simulink model "simulation_nonscalar"  (R2021b)
settings: Solver=VariableStepAuto  StartTime=0.0  StopTime=3  MaxStep=0.005  RelTol=1e-3
values from neighbouring files (symbols this model uses):
  A = round(A,1)    [nonscalar_net.m]    (also in scalar.mat = [-1.7 0 0 0 0 0 -4.8 0 0 0 0 0 ... (25 elements, 5x5)]; scalar_net.m; scalar_net_CreationNewConnection.m = diag([-1,-3,-2]); scalar_net_exception1.m)
  M = [-1.5 0 -0.7 0 17.9 0 -4.1 -6.8 0 0 0 0 ... (25 elements, 5x5)]    [exception.mat]    (also in nonscalar.mat = [-3.8 1.9 -4.5 0 0 0 -4.6 1.6 0 0 0 0 ... (25 elements, 5x5); nonscalar_net.m = round(M,1); nonscalar_net_general.m = sym('M',sum(n)); robustness.mat = [-8.5 0 -1.6 0 1.5 0 -5.3 -4.7 0 0 0 0 ... (25 elements, 5x5)
  M_bar = [-8.5 0 -1.6 0 2.22044604925e-16 0 -5.3 -4.7 0 0 0 0 ... (25 elements, 5x5)]    [robustness.mat]    (also in scalar.mat = [-1.7 0 -6.4 0 0.05 0 -4.8 -9.5 0 0 0 0 ... (25 elements, 5x; test_meerkov_nonscalar_different.m = M + B_bar; test_meerkov_nonscalar_equal.m = M + V_bar)
  mu = sqrt(abs(2/(M(4,5)*M(5,4))))*omega    [nonscalar_net.m]
  n = 1    [exception.mat]    (also in nonscalar_net.m = [1,3,1]; nonscalar_net_general.m = [1,1,1,1]; random.m; robustness.mat)
  omega = 200    [nonscalar.mat]    (also in nonscalar_net.m = 50)
  x_0 = [1 1 1 1 1]    [exception.mat]    (also in nonscalar_net.m = ones(sum(n),1); robustness.mat; scalar.mat; scalar_net.m = ones(5,1))
  y_0 = double(inv_F0*x_0)    [nonscalar_net.m]    (also in scalar_net.m)
settings Model: Creator=alber  LastModifiedBy=alber

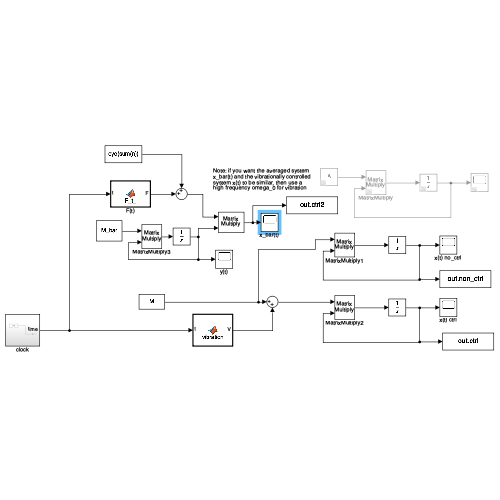
[thumbnail: Simulink's stored preview of the top-level diagram]
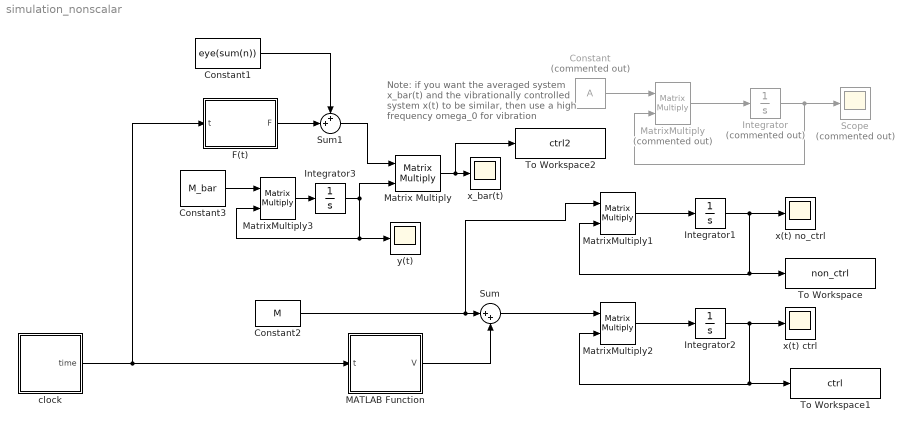
== system simulation_nonscalar ==
  note: Note: if you want the averaged system x_bar(t) and the vibrationally controlled system x(t) to be similar, then use a high frequency omega_0 for vibration
  Constant : Constant  Commented=on  Value=A
  Constant1 : Constant  Value=eye(sum(n))
  Constant2 : Constant  Value=M
  Constant3 : Constant  Value=M_bar
  F(t) : MATLAB Function  TreatAsAtomicUnit=on
  Integrator : Integrator  Commented=on  InitialCondition=x_0
  Integrator1 : Integrator  InitialCondition=x_0
  Integrator2 : Integrator  InitialCondition=x_0
  Integrator3 : Integrator  InitialCondition=y_0
  MATLAB Function : MATLAB Function  TreatAsAtomicUnit=on
  Matrix Multiply : Product  Multiplication=Matrix(*)
  MatrixMultiply : Product  Commented=on  Multiplication=Matrix(*)
  MatrixMultiply1 : Product  Multiplication=Matrix(*)
  MatrixMultiply2 : Product  Multiplication=Matrix(*)
  MatrixMultiply3 : Product  Multiplication=Matrix(*)
  Scope : Scope  Commented=on
  Sum : Sum  Inputs=|++
  Sum1 : Sum  Inputs=++|
  To Workspace : ToWorkspace  VariableName=non_ctrl  SaveFormat=Timeseries  SampleTime=-1
  To Workspace1 : ToWorkspace  VariableName=ctrl  SaveFormat=Timeseries  SampleTime=-1
  To Workspace2 : ToWorkspace  VariableName=ctrl2  SaveFormat=Timeseries  SampleTime=-1
  clock : Subsystem
  x(t) ctrl : Scope
  x(t) no_ctrl : Scope
  x_bar(t) : Scope
  y(t) : Scope
  wires:
  Constant/1 -> MatrixMultiply/1
  Integrator/1 -> Scope/1, MatrixMultiply/2
  MatrixMultiply/1 -> Integrator/1
  MatrixMultiply1/1 -> Integrator1/1
  Constant2/1 -> MatrixMultiply1/1, Sum/1
  Integrator1/1 -> x(t) no_ctrl/1, MatrixMultiply1/2, To Workspace/1
  Integrator2/1 -> x(t) ctrl/1, To Workspace1/1, MatrixMultiply2/2
  MatrixMultiply2/1 -> Integrator2/1
  Sum/1 -> MatrixMultiply2/1
  MATLAB Function/1(V) -> Sum/2
  Constant3/1 -> MatrixMultiply3/1
  MatrixMultiply3/1 -> Integrator3/1
  Integrator3/1 -> Matrix Multiply/2, MatrixMultiply3/2, y(t)/1
  Matrix Multiply/1 -> To Workspace2/1, x_bar(t)/1
  clock/1(time) -> F(t)/1(t), MATLAB Function/1(t)
  F(t)/1(F) -> Sum1/2
  Constant1/1 -> Sum1/1
  Sum1/1 -> Matrix Multiply/1

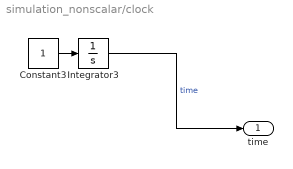
== system simulation_nonscalar/clock ==
  Constant3 : Constant
  Integrator3 : Integrator
  time : Outport
  wires:
  Constant3/1 -> Integrator3/1
  Integrator3/1 -> time/1  "time"

== matlab function simulation_nonscalar/MATLAB Function ==
  data: t input; V output; omega parameter; mu parameter; M parameter
function V = vibration(t, omega, mu, M)

V = zeros(5);
V(5,3) = mu*M(5,3)*sin(omega*t);
V(5,4) = mu*M(5,4)*sin(omega*t);

== matlab function simulation_nonscalar/F(t) ==
  data: t input; F output
function F = F_t_(t)
%#codegen

%    This function was generated by the Symbolic Math Toolbox version 9.0.
%    07-Jun-2023 23:43:06

t2 = t.*5.0e+1;
t4 = sqrt(7.0);
t3 = cos(t2);
F = reshape([0.0,0.0,0.0,0.0,0.0,0.0,0.0,0.0,0.0,0.0,0.0,0.0,0.0,0.0,t3.*t4.*(-8.7e+1./1.54e+2),0.0,0.0,0.0,0.0,t3.*t4.*(-1.0./2.0),0.0,0.0,0.0,0.0,0.0],[5,5]);
